simulink subsystem "single_veh_in_fleet_subsystem"  (R2025b)
settings: Solver=VariableStepAuto  StartTime=0.0  StopTime=10.0  RelTol=1e-3
settings Model: Creator=admin  LastModifiedBy=admin

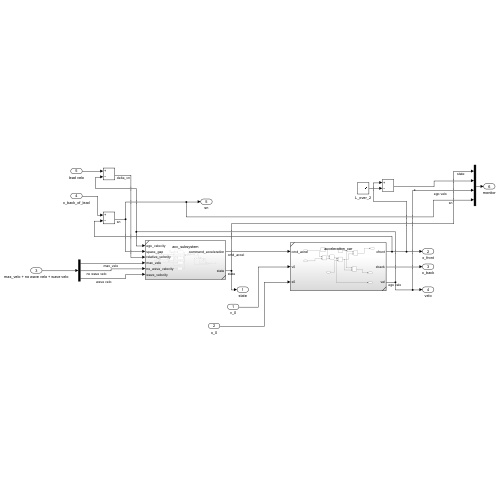
[thumbnail: Simulink's stored preview of the top-level diagram]
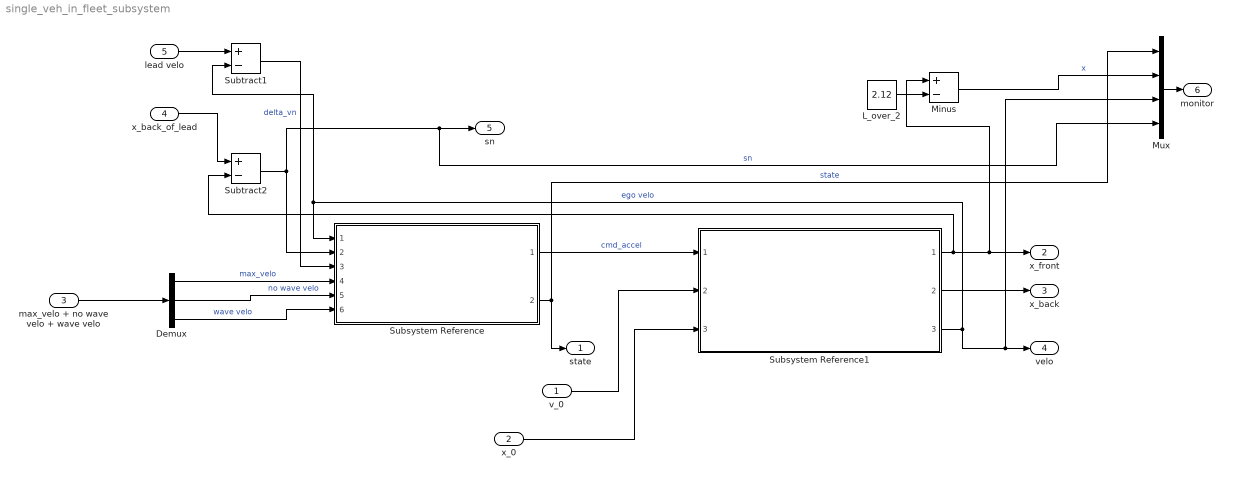
== system single_veh_in_fleet_subsystem ==
  v_0 : Inport
  x_0 : Inport  Port=2
  max_velo + no wave velo + wave velo : Inport  Port=3
  x_back_of_lead : Inport  Port=4
  lead velo : Inport  Port=5
  Demux : Demux  Outputs=3
  L_over_2 : Constant  Value=2.12
  Minus : Sum  Inputs=+-
  Mux : Mux
  Subsystem Reference : Subsystem  ReferencedSubsystem=acc_subsystem
  Subsystem Reference1 : Subsystem  ReferencedSubsystem=acceleration_car
  Subtract1 : Sum  Inputs=+-
  Subtract2 : Sum  Inputs=+-
  state : Outport
  x_front : Outport  Port=2
  x_back : Outport  Port=3
  velo : Outport  Port=4
  sn : Outport  Port=5
  monitor : Outport  Port=6
  wires:
  Subsystem Reference/1 -> Subsystem Reference1/1  "cmd_accel"
  v_0/1 -> Subsystem Reference1/2
  Subsystem Reference1/3 -> Subtract1/2, Subsystem Reference/1, Mux/3, velo/1  "ego velo"
  Subsystem Reference/2 -> state/1, Mux/1  "state"
  Subsystem Reference1/1 -> Subtract2/2, Minus/1, x_front/1
  Subsystem Reference1/2 -> x_back/1
  x_back_of_lead/1 -> Subtract2/1
  Subtract2/1 -> Subsystem Reference/2, Mux/4, sn/1  "sn"
  lead velo/1 -> Subtract1/1
  Subtract1/1 -> Subsystem Reference/3  "delta_vn"
  x_0/1 -> Subsystem Reference1/3
  Demux/1 -> Subsystem Reference/4  "max_velo"
  Demux/2 -> Subsystem Reference/5  "no wave velo"
  Demux/3 -> Subsystem Reference/6  "wave velo"
  max_velo + no wave velo + wave velo/1 -> Demux/1
  L_over_2/1 -> Minus/2
  Minus/1 -> Mux/2  "x"
  Mux/1 -> monitor/1
